simulink model "pedal"  (R2022b)
settings: Solver=VariableStepAuto  StartTime=0.0  StopTime=10.0  RelTol=1e-3
settings Model: Creator=Pietro  LastModifiedBy=Pietro

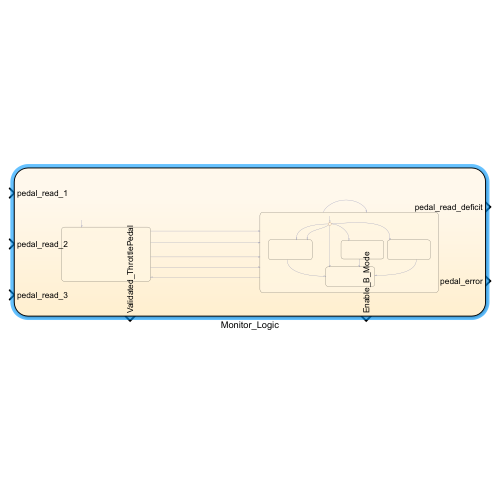
[thumbnail: Simulink's stored preview of the top-level diagram]
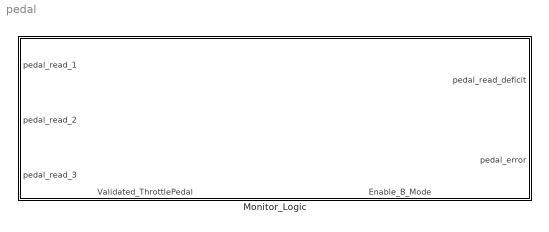
== system pedal ==
  Monitor_Logic : Stateflow chart  TreatAsAtomicUnit=on
      settings: PortSchema="{\"entries\":[{\"content\":{\"sides\":[{\"content\":{\"connectorIds\":[\"In1\",\"In2\",\"In3\"]},\"type\":\"ConnectorPlacement.EquallySpacedRectSide\",\"uuid\":\"7e8062ab-7569-4291-8a74-652e83b32fc9\"},{\"content\":{\"connectorIds\":[\"Out4\",\"Out1\"],\"side\":\"RIGHT\"},\"type\":\"ConnectorPlacement.EquallySpacedRectSide\",\"uuid\":\"87055ce6-60fb-4f5d-a4ce-509dd03ecabb\"},{\"content\":{\"connectorIds\":[],\"side\":\"TOP\"},\"type\":\"ConnectorPlacement.EquallySpacedRectSide\",\"uuid\":\"664d0b31-195e-4c3a-800d-28edce825c84\"},{\"content\":{\"connectorIds\":[\"Out3\",\"Out2\"],\"side\":\"BOTTOM\"},\"type\":\"ConnectorPlacement.EquallySpacedRectSide\",\"uuid\":\"dba6af62-ac30-49a2-a268-36ec45fb9dc4\"}]},\"type\":\"ConnectorPlacement.EquallySpacedConnector\",\"uuid\":\"f578971b-a210-44ee-957a-32c0f6c1d097\"}],\"packageUris\":[\"http://schema.mathworks.com/mf0/Connector/R2020b\"],\"version\":\"1.0\"}"

== stateflow chart pedal/Monitor_Logic ==
  state Fault_mode
    entry:
    Enable_B_Mode = false
    state pedal_read_1_wrong
      entry:
      pedal_read_deficit = true
      during:
      Validated_ThrottlePedal =...
      (pedal_read_2+pedal_read_3)/2
    state pedal_read_3_wrong
      entry:
      pedal_read_deficit = true
      during:
      Validated_ThrottlePedal =...
      (pedal_read_2+pedal_read_1)/2
    state pedal_read_2_wrong
      entry:
      pedal_read_deficit = true
      during:
      Validated_ThrottlePedal =...
      (pedal_read_1+pedal_read_3)/2
    state No_pedal_read
      entry:
      pedal_error = true;
    (default) -> (junction 66)
    (junction 66) -> pedal_read_3_wrong [order 2] : [Flag == 3]
    (junction 66) -> pedal_read_1_wrong [order 5]
    (junction 66) -> pedal_read_2_wrong [order 4] : [Flag == 2]
    (junction 66) -> pedal_read_1_wrong [order 1] : [Flag == 1]
    (junction 66) -> No_pedal_read [order 3] : [Flag == 4]
    pedal_read_2_wrong -> No_pedal_read : [Flag == 4]
    pedal_read_3_wrong -> No_pedal_read : [Flag == 4]
    pedal_read_1_wrong -> No_pedal_read : [Flag == 4]
  state Normal_mode
    entry:
    pedal_read_deficit = false
    pedal_error=false
    Enable_B_Mode = true
    Flag = -1
    during:
    Validated_ThrottlePedal = (pedal_read_1 + pedal_read_2 + pedal_read_3)/3
  Fault_mode -> Fault_mode [order 2] : [abs(pedal_read_1-pedal_read_2)  >= 0.01 && abs(pedal_read_2-pedal_read_3)  >= 0.01...
      |  && abs(pedal_read_1-pedal_read_3) >= 0.01 && Flag ~= 4]{Flag = 4}
  (default) -> Normal_mode
  Normal_mode -> Fault_mode [order 2] : [abs(pedal_read_1-pedal_read_2)  >= 0.01 &&...
      |  abs(pedal_read_1-pedal_read_3) >= 0.01 &&...
      |  abs(pedal_read_2-pedal_read_3) < 0.01]{Flag = 1}
  Normal_mode -> Fault_mode [order 3] : [abs(pedal_read_1-pedal_read_2)  >= 0.01 &&...
      |  abs(pedal_read_2-pedal_read_3) >= 0.01 &&...
      |  abs(pedal_read_1-pedal_read_3) < 0.01]{Flag = 2}
  Normal_mode -> Fault_mode [order 4] : [abs(pedal_read_1-pedal_read_3)  >= 0.01 &&...
      |  abs(pedal_read_2-pedal_read_3) >= 0.01 &&...
      |  abs(pedal_read_1-pedal_read_2) < 0.01]{Flag = 3}
  Normal_mode -> Fault_mode [order 1] : [abs(pedal_read_1-pedal_read_2)  >= 0.01 && abs(pedal_read_2-pedal_read_3)  >= 0.01...
      |  && abs(pedal_read_1-pedal_read_3) >= 0.01]{Flag = 4}
  Fault_mode -> Normal_mode [order 1] : [ abs(pedal_read_1-pedal_read_2)  < 0.01 &&  abs(pedal_read_2-pedal_read_3)  < 0.01 ]
  data: pedal_error output; Enable_B_Mode output; pedal_read_1 input; pedal_read_2 input; pedal_read_3 input; Validated_ThrottlePedal output; Flag local; pedal_read_deficit output
